simulink model "UAV_GCS_Threat_Link"  (R2026a)
settings: Solver=FixedStepDiscrete  StopTime=0.01
libraries: commchan3 x1, commrandsrc3 x1
settings Model: Creator=Adi Suliman  LastModifiedBy=Adi Suliman

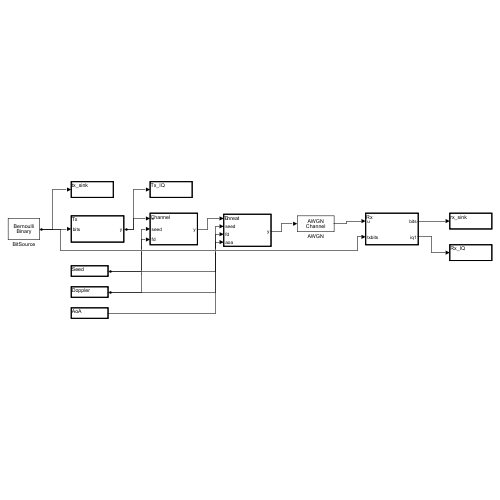
[thumbnail: Simulink's stored preview of the top-level diagram]
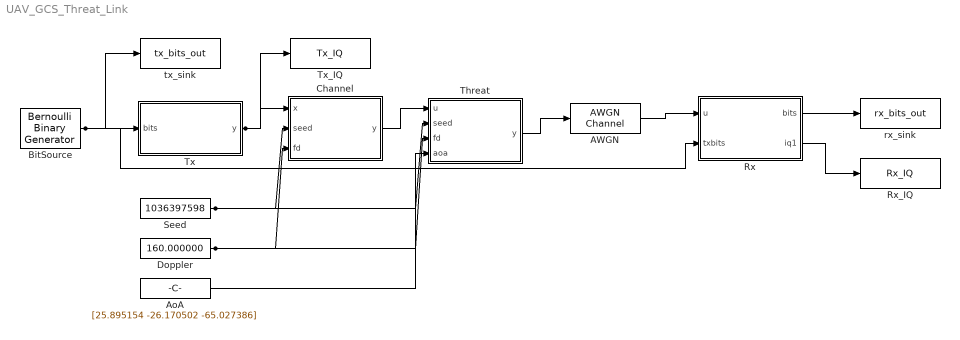
== system UAV_GCS_Threat_Link ==
  AWGN : commchan3/AWGN Channel  LegacyMode=off  NoiseMethod="Signal to noise ratio  (SNR)"  noiseMode="Signal to noise ratio  (SNR)"  EbNo=10  EsNo=10  SNR=-3.0103  BitsPerSymbol=1  SignalPower=0.25  SpecifySymbolPeriod=off  SamplesPerSymbol=1  SymbolPeriod=1  VarianceSource=Parameter  Variance=1  RandomStream=mt19937ar with seed  Seed=1036397599  SimulateUsing=Code generation
  AoA : Constant  Value=[25.895154 -26.170502 -65.027386]
  BitSource : commrandsrc3/Bernoulli Binary Generator  ProbabilityOfZero=0.5  SeedSource=Parameter  Seed=1036397600  SampleTime=5e-07  SamplesPerFrame=1032  OutputDataType=double  SimulateUsing=Interpreted execution
  Channel : MATLAB Function  TreatAsAtomicUnit=on
  Doppler : Constant  Value=160.000000
  Rx : MATLAB Function  TreatAsAtomicUnit=on
  Rx_IQ : ToWorkspace  VariableName=Rx_IQ  SampleTime=-1
  Seed : Constant  Value=1036397598
  Threat : MATLAB Function  TreatAsAtomicUnit=on
  Tx : MATLAB Function  TreatAsAtomicUnit=on
  Tx_IQ : ToWorkspace  VariableName=Tx_IQ  SampleTime=-1
  rx_sink : ToWorkspace  VariableName=rx_bits_out  SampleTime=-1
  tx_sink : ToWorkspace  VariableName=tx_bits_out  SampleTime=-1
  wires:
  BitSource/1 -> Tx/1(bits), Rx/2(txbits), tx_sink/1
  Tx/1(y) -> Channel/1(x), Tx_IQ/1
  Seed/1 -> Channel/2(seed), Threat/2(seed)
  Doppler/1 -> Channel/3(fd), Threat/3(fd)
  AoA/1 -> Threat/4(aoa)
  Channel/1(y) -> Threat/1(u)
  Threat/1(y) -> AWGN/1
  AWGN/1 -> Rx/1(u)
  Rx/1(bits) -> rx_sink/1
  Rx/2(iq1) -> Rx_IQ/1

== matlab function UAV_GCS_Threat_Link/Channel ==
  data: x input; y output; seed input; fd input
function y = fcn(x, seed, fd)
%#codegen
persistent f0 ph n
if isempty(f0)
    rng(seed, 'twister');
end
if isempty(f0)
    f0 = fd * cos(2*pi*rand(32, 2));
end
if isempty(ph)
    ph = 2*pi*rand(32, 2);
end
if isempty(n)
    n = 0;
end
Ns = size(x, 1);
t = (n + (0:Ns-1).') / 4000000.0;
n = n + Ns;
D = complex(zeros(Ns, 2));
for k = 1:2
    D(:, k) = exp(1j * (2*pi*t*f0(:, k).' + repmat(ph(:, k).', Ns, 1))) * ones(32, 1) / sqrt(32);
end
D = D * [1 0.3;0 0.953939201417];
a = [complex(1.000000000000, 0.000000000000); complex(1.000000000000, 0.000000000000)];
y = complex(zeros(Ns, 2));
for k = 1:2
    y(:, k) = x .* (0.9534625892 * a(k) + 0.3015113446 * D(:, k));
end
end

== matlab function UAV_GCS_Threat_Link/Tx ==
  data: bits input; y output
function y = fcn(bits)
%#codegen
persistent txf
if isempty(txf)
    txf = comm.RaisedCosineTransmitFilter('RolloffFactor', 0.250000, 'FilterSpanInSymbols', 10, 'OutputSamplesPerSymbol', 4);
end
sym = pskmod(bits, 4, pi/4, 'gray', 'InputType', 'bit');
y = txf(sym);
end

== matlab function UAV_GCS_Threat_Link/Threat ==
  data: u input; y output; seed input; fd input; aoa input
function y = fcn(u, seed, fd, aoa)
%#codegen
persistent seeded
persistent nI
persistent fI1
persistent pI1
if isempty(seeded)
    seeded = true;
    rng(seed + 7, 'twister');
end
if isempty(nI)
    nI = 0;
end
if isempty(fI1)
    fI1 = fd * cos(2*pi*rand(32, 2));
end
if isempty(pI1)
    pI1 = 2*pi*rand(32, 2);
end
Ns = size(u, 1);
y = u;
t = (nI + (0:Ns-1).') / 4000000.0;
nI = nI + Ns;
ys = y(:, 1);
w = sqrt(0.62797161/2) * complex(randn(Ns, 1), randn(Ns, 1));
dI = complex(zeros(Ns, 2));
for k = 1:2
    dI(:, k) = exp(1j * (2*pi*t*fI1(:, k).' + repmat(pI1(:, k).', Ns, 1))) * ones(32, 1) / sqrt(32);
end
dI = dI * [1 0.3;0 0.953939201417];
aI = exp(-1j * 3.141592653590 * (0:1).' * sind(aoa(1)));
for k = 1:2
    y(:, k) = y(:, k) + w .* (0.9534625892 * aI(k) + 0.3015113446 * dI(:, k));
end
end

== matlab function UAV_GCS_Threat_Link/Rx ==
  data: u input; bits output; txbits input; iq1 output
function [bits, iq1] = fcn(u, txbits)
%#codegen
persistent rxf sbuf
NR = 2; SPS = 4; Dt = 10; B = 64; MODE = 1;
if isempty(rxf)
    rxf = comm.RaisedCosineReceiveFilter('RolloffFactor', 0.250000, 'FilterSpanInSymbols', 10, 'InputSamplesPerSymbol', SPS, 'DecimationFactor', SPS);
end
if isempty(sbuf)
    sbuf = complex(zeros(Dt, 1));
end
iq1 = u(:, 1);
r = rxf(u);
Nsym = size(r, 1);
st = pskmod(txbits, 4, pi/4, 'gray', 'InputType', 'bit');
sa = [sbuf; st(1:Nsym-Dt)];
sbuf = st(Nsym-Dt+1:Nsym);
z = complex(zeros(Nsym, 1));
nb = ceil(Nsym / B);
for bi = 1:nb
    i0 = (bi-1)*B + 1; i1 = min(bi*B, Nsym); n = i1 - i0 + 1;
    h = complex(zeros(NR, 1));
    es = 0;
    for m = i0:i1
        h = h + r(m, :).' * conj(sa(m));
        es = es + abs(sa(m))^2;
    end
    hs = h;
    h = h / max(es, 1e-12);
    Ri = complex(eye(NR));
    if MODE == 2
        R = complex(zeros(NR, NR));
        for m = i0:i1
            e = r(m, :).' - h * sa(m);
            R = R + e * e';
        end
        R = R / n;
        R = R + (1e-3 * real(trace(R)) / NR + 1e-12) * eye(NR);
        Ri = inv(R);
    end
    for m = i0:i1
        hm = (hs - r(m, :).' * conj(sa(m))) / max(es - abs(sa(m))^2, 1e-12);
        w = Ri * hm;
        z(m) = w' * r(m, :).';
    end
end
bits = pskdemod(z, 4, pi/4, 'gray', 'OutputType', 'bit');
end
